simulink model "DC_model_2014a"  (R2014a)
settings: Solver=ode45  StartTime=0.0  StopTime=10.0  MaxStep=0.0001  RelTol=1e-3
values from neighbouring files (symbols this model uses):
  b = 0.2    [Data.mat]
  j = 0.01    [Data.mat]
  K = 0.1    [Data.mat]
  L = 0.5    [Data.mat]
  R = 1    [Data.mat]
  Vs = 100    [Data.mat]
undefined symbols (not defined in the file or in its folder): sigbuilder_block
libraries: simulink x1
settings Model: Creator=maboelfo  LastModifiedBy=HP
settings DebuggingCC: MergeDetectMultiDrivingBlocksExec=error

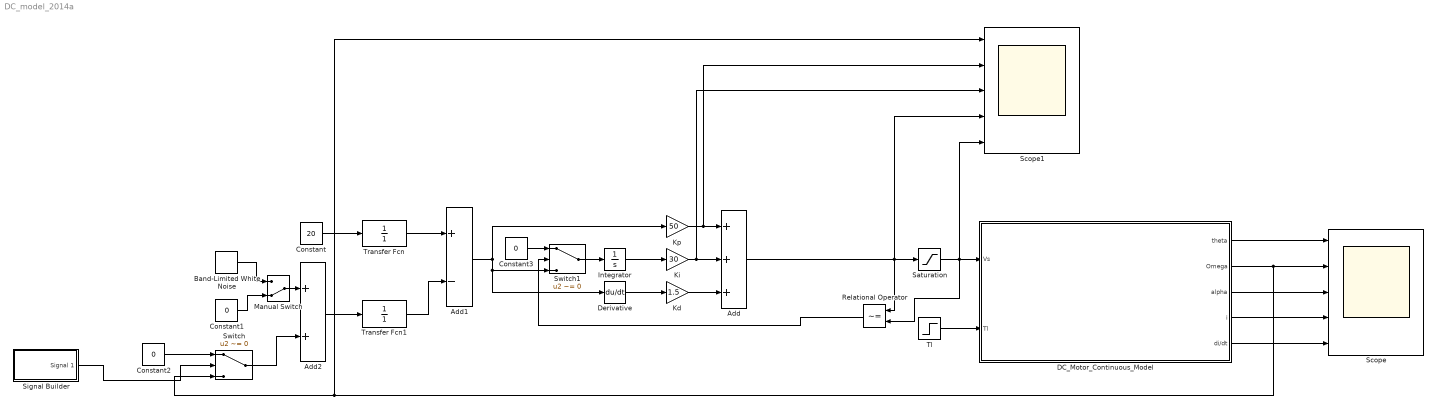
== system DC_model_2014a ==
  Add : Sum  Inputs=+++
  Add1 : Sum  Inputs=+-
  Add2 : Sum
  Band-Limited White Noise : simulink/Sources/Band-Limited White Noise  Cov=[0.0001]  Ts=0.001  seed=[23341]
  Constant : Constant  Value=20
  Constant1 : Constant  Value=0
  Constant2 : Constant  Value=0
  Constant3 : Constant  Value=0
  DC_Motor_Continuous_Model : Subsystem
  Derivative : Derivative
  Integrator : Integrator
  Kd : Gain  Gain=1.5
  Ki : Gain  Gain=30
  Kp : Gain  Gain=50
  Manual Switch : ManualSwitch  CurrentSetting=0
  Relational Operator : RelationalOperator  Operator=~=  OutDataTypeStr=boolean
  Saturation : Saturate  UpperLimit=Vs  LowerLimit=0
  Scope : Scope  NumInputPorts=5
      settings: YMin=-5~-5~-5~-5~-5  YMax=5~5~5~5~5
  Scope1 : Scope  NumInputPorts=5
      settings: YMin=-5~-5~-5~-5~-5  YMax=5~5~5~5~5
  Signal Builder : Subsystem  Tag=STV Subsys  LoadFcn=sigbuilder_block('load');  StartFcn=sigbuilder_block('start');  StopFcn=sigbuilder_block('stop');  ClipboardFcn=sigbuilder_block('clipboard');  mask(Sigbuilder block){}
      mask help: Simulink:masks:SigbuilderBlock_MD
      mask init:
      | if ~strcmp(get_param(bdroot(gcbh),'SimulationStatus'),'stopped') tuvar = sigbuilder_block('maskInit'); end
      settings: CopyFcn=sigbuilder_block('copy');  DeleteFcn=sigbuilder_block('delete');  ModelCloseFcn=sigbuilder_block('modelClose');  PreSaveFcn=sigbuilder_block('preSave');  PauseFcn=sigbuilder_block('pause');  ContinueFcn=sigbuilder_block('continue');  NameChangeFcn=sigbuilder_block('namechange');  OpenFcn=sigbuilder_block('open',[437.25 180 550.5 395.25 ]);  CloseFcn=sigbuilder_block('close');
      mask Display: plot(0, 0, 100, 100,[2, 2, 32, 32, 2], [68, 8, 8, 68, 68],[32, 2], [38, 38], [32, 19, 2],[53, 60, 44], [32, 17, 17, 2],[16, 16, 31, 31]);txt = getActiveGroup(gcbh);text(2, 100, txt,'verticalAlignment', 'top');
  Switch : Switch  Criteria=u2 ~= 0
  Switch1 : Switch  Criteria=u2 ~= 0
  Tl : Step  Time=5  SampleTime=0
  Transfer Fcn : TransferFcn  Denominator=[1]
  Transfer Fcn1 : TransferFcn  Denominator=[1]
  wires:
  Kp/1 -> Scope1/2, Add/1
  Ki/1 -> Add/2, Scope1/3
  Kd/1 -> Add/3
  Add/1 -> Relational Operator/1, Scope1/4, Saturation/1
  Integrator/1 -> Ki/1
  Derivative/1 -> Kd/1
  Add1/1 -> Switch1/3, Derivative/1, Kp/1
  DC_Motor_Continuous_Model/2(Omega) -> Switch/3, Scope1/1, Scope/2
  Tl/1 -> DC_Motor_Continuous_Model/2(Tl)
  Constant/1 -> Transfer Fcn/1
  DC_Motor_Continuous_Model/1(theta) -> Scope/1
  DC_Motor_Continuous_Model/3(alpha) -> Scope/3
  DC_Motor_Continuous_Model/4(i) -> Scope/4
  DC_Motor_Continuous_Model/5(di/dt) -> Scope/5
  Transfer Fcn/1 -> Add1/1
  Add2/1 -> Transfer Fcn1/1
  Constant1/1 -> Manual Switch/2
  Manual Switch/1 -> Add2/1
  Band-Limited White Noise/1 -> Manual Switch/1
  Saturation/1 -> Relational Operator/2, Scope1/5, DC_Motor_Continuous_Model/1(Vs)
  Transfer Fcn1/1 -> Add1/2
  Switch/1 -> Add2/2
  Constant2/1 -> Switch/1
  Signal Builder/1(Signal 1) -> Switch/2
  Switch1/1 -> Integrator/1
  Relational Operator/1 -> Switch1/2
  Constant3/1 -> Switch1/1

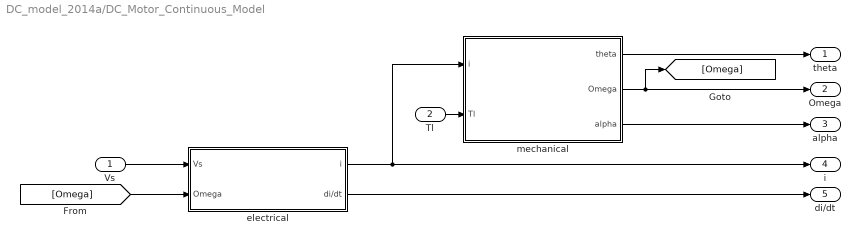
== system DC_model_2014a/DC_Motor_Continuous_Model ==
  Vs : Inport
  Tl : Inport  Port=2
  electrical : Subsystem
  mechanical : Subsystem
  theta : Outport
  Omega : Outport  Port=2
  alpha : Outport  Port=3
  i : Outport  Port=4
  di/dt : Outport  Port=5
  wires:
  Vs/1 -> electrical/1(Vs)
  mechanical/1(theta) -> theta/1
  [Omega] -> electrical/2(Omega)
  mechanical/2(Omega) -> Omega/1, [Omega]
  Tl/1 -> mechanical/2(Tl)
  electrical/1(i) -> i/1, mechanical/1(i)
  electrical/2(di/dt) -> di/dt/1
  mechanical/3(alpha) -> alpha/1

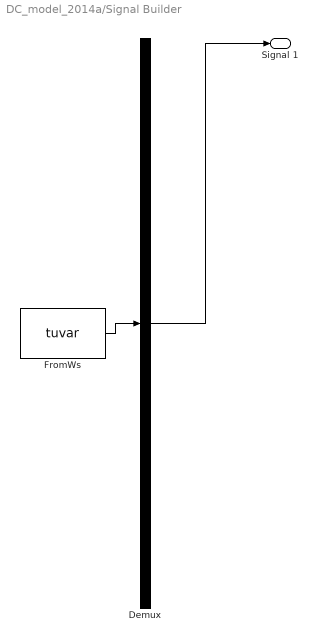
== system DC_model_2014a/Signal Builder ==
  Demux : Demux  Tag=STV Demux  Outputs=1
  FromWs : FromWorkspace  Tag=STV FromWs  VariableName=tuvar  SampleTime=0
      SigBuilderData=|
      | common.afterFinalStr = 'Extrapolate'
      | common.sampleTime = 0
      | dataSet.timeRange = [0 10]
      | dataSet.name = 'Group 1'
      | sbobj.Groups.Name = 'Group 1'
      | sbobj.Groups.Signals.Name = 'Signal 1'
      | sbobj.Groups.Signals.XData = [0 1 1 6 6 10]
      | sbobj.Groups.Signals.YData = [0 0 1 1 0 0]
  Signal 1 : Outport  Tag=STV Outport
  wires:
  Demux/1 -> Signal 1/1
  FromWs/1 -> Demux/1

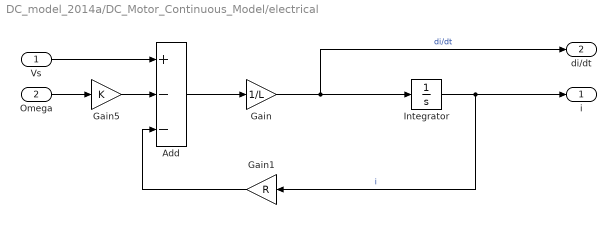
== system DC_model_2014a/DC_Motor_Continuous_Model/electrical ==
  Vs : Inport
  Omega : Inport  Port=2
  Add : Sum  Inputs=+--
  Gain : Gain  Gain=1/L
  Gain1 : Gain  Gain=R
  Gain5 : Gain  Gain=K
  Integrator : Integrator
  i : Outport
  di/dt : Outport  Port=2
  wires:
  Gain/1 -> di/dt/1, Integrator/1  "di/dt"
  Gain1/1 -> Add/3
  Integrator/1 -> i/1, Gain1/1  "i"
  Add/1 -> Gain/1
  Vs/1 -> Add/1
  Omega/1 -> Gain5/1
  Gain5/1 -> Add/2

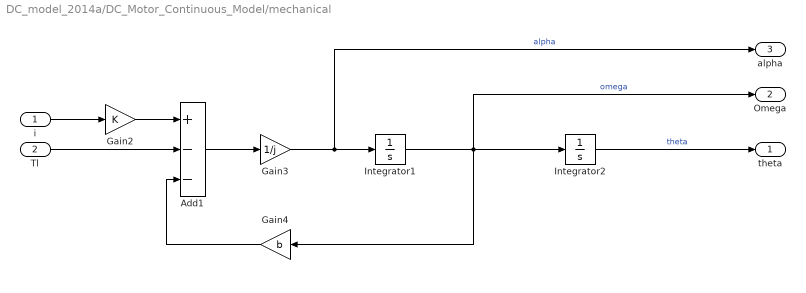
== system DC_model_2014a/DC_Motor_Continuous_Model/mechanical ==
  i : Inport
  Tl : Inport  Port=2
  Add1 : Sum  Inputs=+--
  Gain2 : Gain  Gain=K
  Gain3 : Gain  Gain=1/j
  Gain4 : Gain  Gain=b
  Integrator1 : Integrator
  Integrator2 : Integrator
  theta : Outport
  Omega : Outport  Port=2
  alpha : Outport  Port=3
  wires:
  i/1 -> Gain2/1
  Gain3/1 -> alpha/1, Integrator1/1  "alpha"
  Integrator1/1 -> Omega/1, Gain4/1, Integrator2/1  "omega"
  Integrator2/1 -> theta/1  "theta"
  Gain4/1 -> Add1/3
  Add1/1 -> Gain3/1
  Gain2/1 -> Add1/1
  Tl/1 -> Add1/2
